simulink library "asr"  (Simulink 8.1)
settings: Solver=ode45  StartTime=0.0  StopTime=10.0  RelTol=1e-3
undefined symbols (not defined in the file): FALSE, KJUD_AEBMaxActSpeed_mps, KJUD_AEBMaxDeactSpeed_mps, KJUD_AEBMinActSpeed_mps, KJUD_AEBMinDeactSpeed_mps, TRUE
settings Model: Creator=AT015086  LastModifiedBy=tescamilla

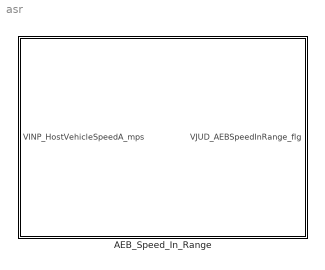
== system asr ==
  AEB_Speed_In_Range : Subsystem

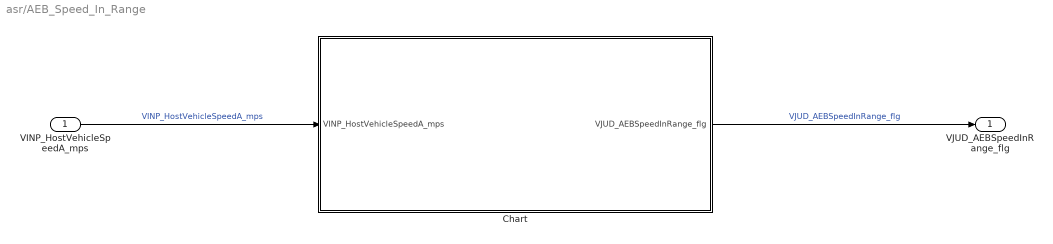
== system asr/AEB_Speed_In_Range ==
  "VINP_HostVehicleSpeedA_mps " : Inport
  Chart : Stateflow chart  TreatAsAtomicUnit=on
  VJUD_AEBSpeedInRange_flg : Outport
  wires:
  "VINP_HostVehicleSpeedA_mps "/1 -> Chart/1(VINP_HostVehicleSpeedA_mps)  "VINP_HostVehicleSpeedA_mps"
  Chart/1(VJUD_AEBSpeedInRange_flg) -> VJUD_AEBSpeedInRange_flg/1  "VJUD_AEBSpeedInRange_flg"

== stateflow chart AEB_Speed_In_Range/Chart ==
  state SPEED_OUT_OF_RANGE
    en:
    VJUD_AEBSpeedInRange_flg=FALSE;
  state SPEED_IN_RANGE
    en:
    VJUD_AEBSpeedInRange_flg=TRUE;
  (default) -> SPEED_OUT_OF_RANGE
  SPEED_OUT_OF_RANGE -> SPEED_IN_RANGE : [(VINP_HostVehicleSpeedA_mps>KJUD_AEBMinActSpeed_mps)&&...
      | (VINP_HostVehicleSpeedA_mps<KJUD_AEBMaxActSpeed_mps)]
  SPEED_IN_RANGE -> SPEED_OUT_OF_RANGE : [(VINP_HostVehicleSpeedA_mps<KJUD_AEBMinDeactSpeed_mps)||...
      | (VINP_HostVehicleSpeedA_mps>KJUD_AEBMaxDeactSpeed_mps)]
  data: VINP_HostVehicleSpeedA_mps input single; VJUD_AEBSpeedInRange_flg output boolean; FALSE parameter boolean; TRUE parameter boolean; KJUD_AEBMaxActSpeed_mps parameter single; KJUD_AEBMinActSpeed_mps parameter single; KJUD_AEBMaxDeactSpeed_mps parameter single; KJUD_AEBMinDeactSpeed_mps parameter single
